simulink model "sampleModel1629"  (R2023a)
settings: Solver=VariableStepAuto  StartTime=0.0  StopTime=10.0  RelTol=1e-3
libraries: hdlsllib x8, simulink x2
settings Model: Creator=user1  LastModifiedBy=user1

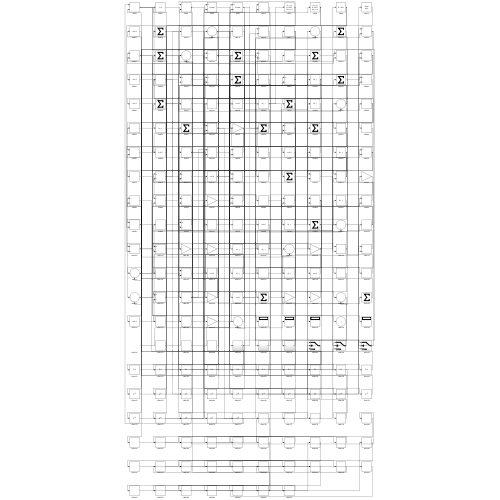
[thumbnail: Simulink's stored preview of the top-level diagram]
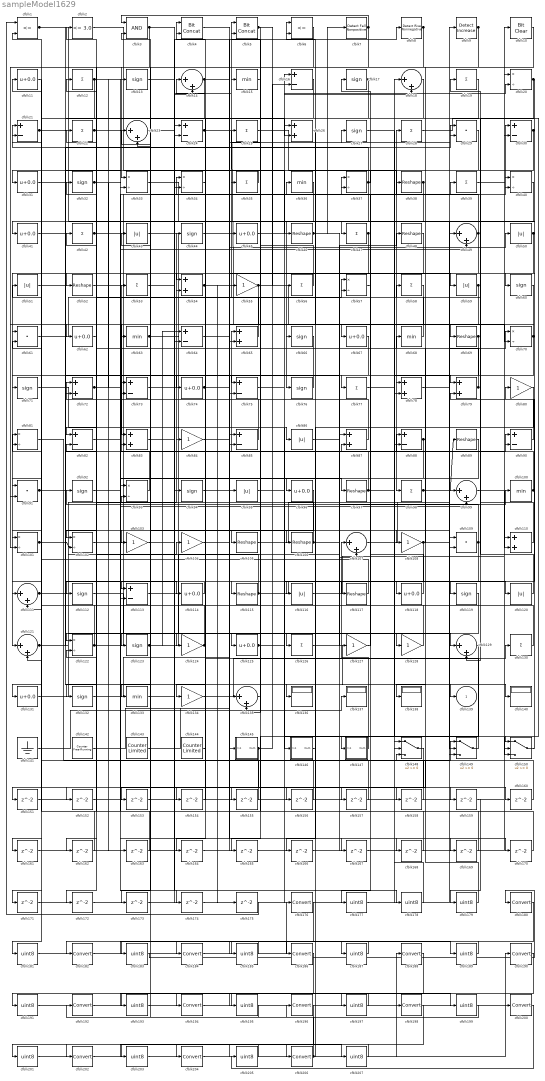
== system sampleModel1629 ==
  cfblk1 : RelationalOperator  Operator=<=  OutDataTypeStr=boolean  InputSameDT=off
  cfblk10 : simulink/Logic and Bit Operations/Bit Clear  iBit=0
      settings: LibrarySourceBlock=|
      | hdlsllib/Logic and Bit
      | Operations/Bit Clear
  cfblk{15,36,63,68,100,133} (6 alike) : MinMax
  cfblk{20,33..34,37,40,57,70,81,93,101..102,122} (12 alike) : Product  Inputs=*/  RndMeth=Zero  SaturateOnIntegerOverflow=on
  cfblk{55,80,84,103..104,108,124,127..128,134} (10 alike) : Gain
  cfblk{38,46,48,52,69,89,97,105..106,115,117} (11 alike) : Reshape
  cfblk{14,18,23,49,99,107,111,121,129,135} (10 alike) : Sum  Inputs=|++
  cfblk{29,61,91,109} (4 alike) : DotProduct  OutDataTypeStr=Inherit: Inherit via internal rule
  cfblk{11,31,41,45,62,67,74,96,114,118,125,131} (12 alike) : Bias  Bias=0.0  SaturateOnIntegerOverflow=off
  cfblk{26,54,65,72,78..79,83,87,110} (9 alike) : Sum
  cfblk{13,17,27,32,44,60,66,71,76,92,94,112,119,123,132} (15 alike) : Signum
  cfblk{16,21,24,30,64,73,75,82,85,88,90,113} (12 alike) : Sum  Inputs=+-
  cfblk{43,50..51,59,86,95,116,120} (8 alike) : Abs  SaturateOnIntegerOverflow=off
  cfblk{12,19,22,25,28,35,39,42,47,53,56,58,77,98,126,130} (16 alike) : Sum  Inputs=+
  cfblk{136..138,140} (4 alike) : Display
  cfblk141 : Ground
  cfblk142 : hdlsllib/Sources/Counter Free-Running  NumBits=16  tsamp=-1
  cfblk143 : hdlsllib/Sources/Counter Limited  uplimit=7  tsamp=-1
  cfblk144 : hdlsllib/Sources/Counter Limited  uplimit=7  tsamp=-1
  cfblk145 : Subsystem
      settings: LibrarySourceBlock=|
      | hdlsllib/Ports &
      | Subsystems/Subsystem
  cfblk146 : Subsystem
      settings: LibrarySourceBlock=|
      | hdlsllib/Ports &
      | Subsystems/Subsystem
  cfblk147 : Subsystem
      settings: LibrarySourceBlock=|
      | hdlsllib/Ports &
      | Subsystems/Subsystem
  cfblk148 : Switch  SaturateOnIntegerOverflow=off  InputSameDT=off
  cfblk149 : Switch  SaturateOnIntegerOverflow=off  InputSameDT=off
  cfblk150 : Switch  SaturateOnIntegerOverflow=off  InputSameDT=off
  cfblk{151..175} (25 alike) : Delay  SampleTime=1
  cfblk{176,180,182,184,186,188,190,192,194,196,198,200,202,204,206} (15 alike) : DataTypeConversion  SaturateOnIntegerOverflow=off  RndMeth=Floor
  cfblk{177..179,181,183,185,187,189,191,193,195,197,199,201,203,205,207} (17 alike) : DataTypeConversion  OutDataTypeStr=uint8  SaturateOnIntegerOverflow=off  RndMeth=Floor
  cfblk2 : hdlsllib/Logic and Bit Operations/Compare To Constant  relop=<=  const=3.0  OutDataTypeStr=boolean
  cfblk3 : Logic  AllPortsSameDT=off  OutDataTypeStr=boolean
  cfblk4 : hdlsllib/Logic and Bit Operations/Bit Concat  numInputs=2
  cfblk5 : hdlsllib/Logic and Bit Operations/Bit Concat  numInputs=2
  cfblk6 : RelationalOperator  Operator=<=  OutDataTypeStr=boolean  InputSameDT=off
  cfblk7 : hdlsllib/Logic and Bit Operations/Detect Fall Nonpositive  vinit=0  OutDataTypeStr=boolean
  cfblk8 : hdlsllib/Logic and Bit Operations/Detect Rise Nonnegative  vinit=0  OutDataTypeStr=boolean
  cfblk9 : simulink/Logic and Bit Operations/Detect Increase  vinit=0.0  OutDataTypeStr=boolean
      settings: LibrarySourceBlock=|
      | hdlsllib/Logic and Bit
      | Operations/Detect
      | Increase
  cfblk139 : Outport  VectorParamsAs1DForOutWhenUnconnected=off
  wires:
  cfblk50/1 -> cfblk121/1, cfblk147/1(In1)
  cfblk54/1 -> cfblk67/1, cfblk175/1
  cfblk100/1 -> cfblk65/1, cfblk43/1
  cfblk49/1 -> cfblk52/1, cfblk23/2, cfblk3/2
  cfblk33/1 -> cfblk119/1
  cfblk134/1 -> cfblk130/1
  cfblk70/1 -> cfblk69/1, cfblk88/2, cfblk173/1
  cfblk47/1 -> cfblk161/1, cfblk162/1
  cfblk65/1 -> cfblk42/1
  cfblk109/1 -> cfblk92/1, cfblk166/1
  cfblk73/1 -> cfblk126/1
  cfblk81/1 -> cfblk149/1
  cfblk41/1 -> cfblk75/1
  cfblk115/1 -> cfblk120/1, cfblk23/1, cfblk72/2
  cfblk3/1 -> cfblk33/1, cfblk159/1
  cfblk1/1 -> cfblk76/1, cfblk103/1, cfblk26/2
  cfblk43/1 -> cfblk86/1
  cfblk111/1 -> cfblk44/1, cfblk29/2
  cfblk80/1 -> cfblk96/1
  cfblk142/1 -> cfblk27/1
  cfblk122/1 -> cfblk30/1, cfblk21/1
  cfblk26/1 -> cfblk66/1
  cfblk29/1 -> cfblk105/1
  cfblk91/1 -> cfblk136/1, cfblk51/1
  cfblk68/1 -> cfblk5/1
  cfblk5/1 -> cfblk115/1, cfblk56/1
  cfblk89/1 -> cfblk116/1
  cfblk28/1 -> cfblk150/1
  cfblk131/1 -> cfblk104/1
  cfblk25/1 -> cfblk98/1
  cfblk22/1 -> cfblk95/1, cfblk99/2
  cfblk34/1 -> cfblk54/1
  cfblk2/1 -> cfblk46/1
  cfblk147/1(Out1) -> cfblk107/1
  cfblk35/1 -> cfblk31/1
  cfblk30/1 -> cfblk121/2, cfblk177/1
  cfblk76/1 -> cfblk74/1
  cfblk12/1 -> cfblk61/1, cfblk97/1
  cfblk7/1 -> cfblk102/1, cfblk91/2, cfblk3/1
  cfblk39/1 -> cfblk40/1
  cfblk85/1 -> cfblk22/1
  cfblk4/1 -> cfblk65/2
  cfblk103/1 -> cfblk6/1
  cfblk123/1 -> cfblk48/1, cfblk64/1, cfblk167/1
  cfblk99/1 -> cfblk110/2
  cfblk24/1 -> cfblk55/1, cfblk168/1
  cfblk79/1 -> cfblk2/1, cfblk57/2
  cfblk125/1 -> cfblk150/2, cfblk18/2
  cfblk72/1 -> cfblk13/1, cfblk169/1
  cfblk116/1 -> cfblk10/1
  cfblk121/1 -> cfblk124/1, cfblk88/1
  cfblk114/1 -> cfblk112/1
  cfblk130/1 -> cfblk81/1
  cfblk94/1 -> cfblk8/1
  cfblk102/1 -> cfblk84/1
  cfblk126/1 -> cfblk140/1
  cfblk120/1 -> cfblk19/1
  cfblk127/1 -> cfblk37/1
  cfblk42/1 -> cfblk28/1, cfblk174/1
  cfblk108/1 -> cfblk68/1, cfblk70/1, cfblk154/1
  cfblk8/1 -> cfblk123/1, cfblk64/2
  cfblk31/1 -> cfblk109/1
  cfblk17/1 -> cfblk41/1, cfblk62/1, cfblk131/1
  cfblk67/1 -> cfblk111/1
  cfblk61/1 -> cfblk45/1
  cfblk55/1 -> cfblk78/1, cfblk63/1
  cfblk95/1 -> cfblk117/1
  cfblk74/1 -> cfblk38/1, cfblk39/1
  cfblk15/1 -> cfblk125/1
  cfblk77/1 -> cfblk79/1
  cfblk53/1 -> cfblk15/1
  cfblk97/1 -> cfblk90/1, cfblk4/2
  cfblk141/1 -> cfblk137/1
  cfblk18/1 -> cfblk134/1
  cfblk104/1 -> cfblk40/2
  cfblk90/1 -> cfblk79/2
  cfblk133/1 -> cfblk87/2
  cfblk64/1 -> cfblk109/2
  cfblk110/1 -> cfblk58/1
  cfblk118/1 -> cfblk34/1
  cfblk16/1 -> cfblk122/1
  cfblk150/1 -> cfblk80/1
  cfblk9/1 -> cfblk82/1, cfblk158/1
  cfblk119/1 -> cfblk132/1
  cfblk75/1 -> cfblk29/1
  cfblk93/1 -> cfblk53/1
  cfblk45/1 -> cfblk20/2
  cfblk60/1 -> cfblk85/2
  cfblk59/1 -> cfblk83/1, cfblk101/2
  cfblk14/1 -> cfblk59/1, cfblk113/1, cfblk70/2
  cfblk46/1 -> cfblk107/2, cfblk7/1
  cfblk32/1 -> cfblk49/2, cfblk163/1
  cfblk107/1 -> cfblk49/1
  cfblk63/1 -> cfblk94/1, cfblk127/1
  cfblk101/1 -> cfblk102/2, cfblk106/1
  cfblk144/1 -> cfblk4/1
  cfblk132/1 -> cfblk75/2
  cfblk82/1 -> cfblk57/1
  cfblk19/1 -> cfblk24/2
  cfblk71/1 -> cfblk146/1(In1)
  cfblk106/1 -> cfblk100/1, cfblk72/1
  cfblk87/1 -> cfblk12/1
  cfblk98/1 -> cfblk89/1, cfblk118/1
  cfblk143/1 -> cfblk50/1
  cfblk21/1 -> cfblk33/2, cfblk114/1
  cfblk37/1 -> cfblk47/1, cfblk17/1, cfblk21/2
  cfblk10/1 -> cfblk128/1
  cfblk58/1 -> cfblk71/1
  cfblk92/1 -> cfblk37/2
  cfblk124/1 -> cfblk83/2, cfblk73/2
  cfblk27/1 -> cfblk149/2
  cfblk83/1 -> cfblk108/1
  cfblk88/1 -> cfblk138/1, cfblk113/2
  cfblk62/1 -> cfblk32/1
  cfblk105/1 -> cfblk9/1
  cfblk38/1 -> cfblk133/1, cfblk78/2
  cfblk6/1 -> cfblk135/2
  cfblk113/1 -> cfblk26/1
  cfblk145/1(Out1) -> cfblk16/2, cfblk152/1
  cfblk149/1 -> cfblk14/1
  cfblk78/1 -> cfblk150/3
  cfblk20/1 -> cfblk60/1, cfblk129/2
  cfblk51/1 -> cfblk139/1
  cfblk117/1 -> cfblk11/1
  cfblk44/1 -> cfblk145/1(In1)
  cfblk66/1 -> cfblk101/1
  cfblk69/1 -> cfblk171/1, cfblk172/1
  cfblk36/1 -> cfblk91/1
  cfblk48/1 -> cfblk77/1
  cfblk146/1(Out1) -> cfblk6/2
  cfblk56/1 -> cfblk35/1
  cfblk135/1 -> cfblk25/1
  cfblk86/1 -> cfblk90/2
  cfblk112/1 -> cfblk129/1
  cfblk128/1 -> cfblk73/1
  cfblk11/1 -> cfblk151/1
  cfblk151/1 -> cfblk20/1
  cfblk152/1 -> cfblk99/1
  cfblk96/1 -> cfblk153/1
  cfblk154/1 -> cfblk54/2
  cfblk52/1 -> cfblk155/1
  cfblk155/1 -> cfblk81/2
  cfblk23/1 -> cfblk156/1
  cfblk156/1 -> cfblk24/1
  cfblk57/1 -> cfblk157/1
  cfblk157/1 -> cfblk82/2
  cfblk158/1 -> cfblk1/2
  cfblk84/1 -> cfblk160/1
  cfblk160/1 -> cfblk85/1
  cfblk161/1 -> cfblk110/1
  cfblk162/1 -> cfblk61/2
  cfblk163/1 -> cfblk93/1
  cfblk40/1 -> cfblk164/1
  cfblk164/1 -> cfblk135/1
  cfblk129/1 -> cfblk165/1
  cfblk165/1 -> cfblk87/1
  cfblk166/1 -> cfblk30/2
  cfblk167/1 -> cfblk18/1
  cfblk168/1 -> cfblk122/2
  cfblk169/1 -> cfblk5/2
  cfblk13/1 -> cfblk170/1
  cfblk170/1 -> cfblk111/2
  cfblk171/1 -> cfblk14/2
  cfblk172/1 -> cfblk34/2
  cfblk173/1 -> cfblk149/3
  cfblk174/1 -> cfblk16/1
  cfblk175/1 -> cfblk1/1
  cfblk177/1 -> cfblk148/1
  cfblk153/1 -> cfblk178/1
  cfblk178/1 -> cfblk148/2
  cfblk159/1 -> cfblk179/1
  cfblk179/1 -> cfblk148/3
  cfblk148/1 -> cfblk181/1
  cfblk181/1 -> cfblk176/1
  cfblk176/1 -> cfblk183/1
  cfblk183/1 -> cfblk180/1
  cfblk180/1 -> cfblk185/1
  cfblk185/1 -> cfblk182/1
  cfblk182/1 -> cfblk187/1
  cfblk187/1 -> cfblk184/1
  cfblk184/1 -> cfblk189/1
  cfblk189/1 -> cfblk186/1
  cfblk186/1 -> cfblk191/1
  cfblk191/1 -> cfblk188/1
  cfblk188/1 -> cfblk193/1
  cfblk193/1 -> cfblk190/1
  cfblk190/1 -> cfblk195/1
  cfblk195/1 -> cfblk192/1
  cfblk192/1 -> cfblk197/1
  cfblk197/1 -> cfblk194/1
  cfblk194/1 -> cfblk199/1
  cfblk199/1 -> cfblk196/1
  cfblk196/1 -> cfblk201/1
  cfblk201/1 -> cfblk198/1
  cfblk198/1 -> cfblk203/1
  cfblk203/1 -> cfblk200/1
  cfblk204/1 -> cfblk206/1
  cfblk200/1 -> cfblk205/1
  cfblk205/1 -> cfblk202/1
  cfblk206/1 -> cfblk93/2, cfblk36/1
  cfblk202/1 -> cfblk207/1
  cfblk207/1 -> cfblk204/1

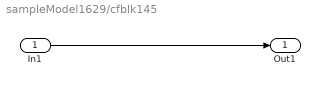
== system sampleModel1629/cfblk145 ==
  In1 : Inport
  Out1 : Outport
  wires:
  In1/1 -> Out1/1

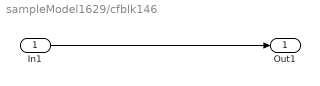
== system sampleModel1629/cfblk146 ==
  In1 : Inport
  Out1 : Outport
  wires:
  In1/1 -> Out1/1

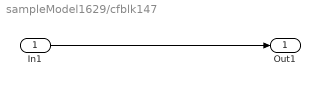
== system sampleModel1629/cfblk147 ==
  In1 : Inport
  Out1 : Outport
  wires:
  In1/1 -> Out1/1
